simulink model "cog"  (R2025b)
settings: Solver=FixedStepAuto  StartTime=0.0  StopTime=10.0  FixedStep=0.01  RelTol=1e-3
libraries: matrix_library x3, SignalEditorBlockLib x1
settings Model: Creator=12482  LastModifiedBy=12482

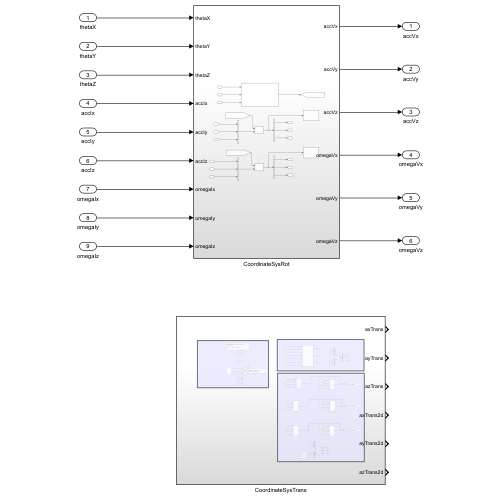
[thumbnail: Simulink's stored preview of the top-level diagram]
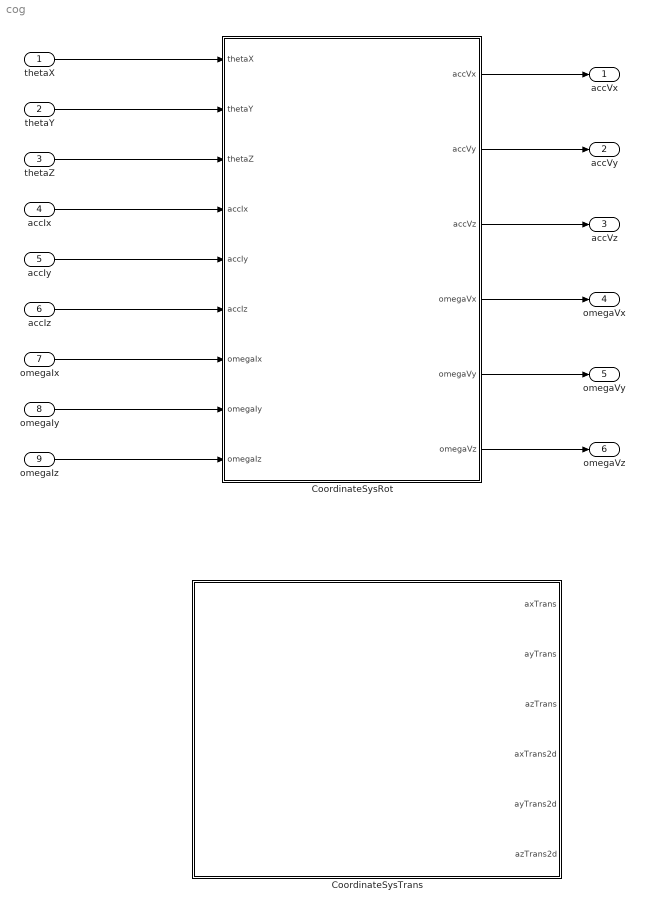
== system cog ==
  thetaX : Inport
  thetaY : Inport  Port=2
  thetaZ : Inport  Port=3
  accIx : Inport  Port=4
  accIy : Inport  Port=5
  accIz : Inport  Port=6
  omegaIx : Inport  Port=7
  omegaIy : Inport  Port=8
  omegaIz : Inport  Port=9
  CoordinateSysRot : Subsystem
  CoordinateSysTrans : Subsystem
  accVx : Outport
  accVy : Outport  Port=2
  accVz : Outport  Port=3
  omegaVx : Outport  Port=4
  omegaVy : Outport  Port=5
  omegaVz : Outport  Port=6
  wires:
  thetaX/1 -> CoordinateSysRot/1(thetaX)
  thetaY/1 -> CoordinateSysRot/2(thetaY)
  thetaZ/1 -> CoordinateSysRot/3(thetaZ)
  accIx/1 -> CoordinateSysRot/4(accIx)
  accIy/1 -> CoordinateSysRot/5(accIy)
  accIz/1 -> CoordinateSysRot/6(accIz)
  omegaIx/1 -> CoordinateSysRot/7(omegaIx)
  omegaIy/1 -> CoordinateSysRot/8(omegaIy)
  omegaIz/1 -> CoordinateSysRot/9(omegaIz)
  CoordinateSysRot/1(accVx) -> accVx/1
  CoordinateSysRot/2(accVy) -> accVy/1
  CoordinateSysRot/3(accVz) -> accVz/1
  CoordinateSysRot/4(omegaVx) -> omegaVx/1
  CoordinateSysRot/5(omegaVy) -> omegaVy/1
  CoordinateSysRot/6(omegaVz) -> omegaVz/1

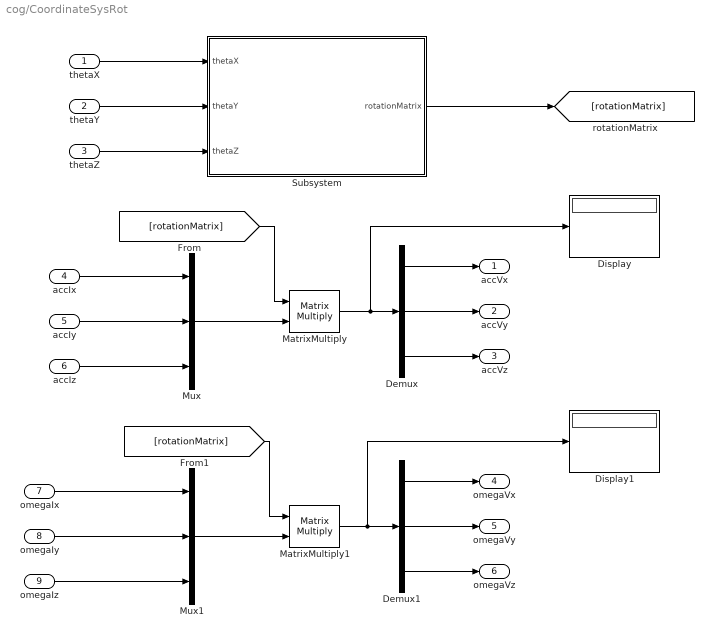
== system cog/CoordinateSysRot ==
  thetaX : Inport
  thetaY : Inport  Port=2
  thetaZ : Inport  Port=3
  accIx : Inport  Port=4
  accIy : Inport  Port=5
  accIz : Inport  Port=6
  omegaIx : Inport  Port=7
  omegaIy : Inport  Port=8
  omegaIz : Inport  Port=9
  Demux : Demux  Outputs=3
  Demux1 : Demux  Outputs=3
  Display : Display
  Display1 : Display
  MatrixMultiply : Product  Multiplication=Matrix(*)
  MatrixMultiply1 : Product  Multiplication=Matrix(*)
  Mux : Mux  Inputs=3
  Mux1 : Mux  Inputs=3
  Subsystem : Subsystem
  accVx : Outport
  accVy : Outport  Port=2
  accVz : Outport  Port=3
  omegaVx : Outport  Port=4
  omegaVy : Outport  Port=5
  omegaVz : Outport  Port=6
  wires:
  thetaX/1 -> Subsystem/1(thetaX)
  Demux1/3 -> omegaVz/1
  accIz/1 -> Mux/3
  Mux/1 -> MatrixMultiply/2
  thetaY/1 -> Subsystem/2(thetaY)
  MatrixMultiply/1 -> Display/1, Demux/1
  Subsystem/1(rotationMatrix) -> [rotationMatrix]
  thetaZ/1 -> Subsystem/3(thetaZ)
  Demux1/1 -> omegaVx/1
  accIx/1 -> Mux/1
  Demux1/2 -> omegaVy/1
  Demux/1 -> accVx/1
  accIy/1 -> Mux/2
  Demux/3 -> accVz/1
  Mux1/1 -> MatrixMultiply1/2
  [rotationMatrix] -> MatrixMultiply1/1
  omegaIx/1 -> Mux1/1
  omegaIy/1 -> Mux1/2
  MatrixMultiply1/1 -> Display1/1, Demux1/1
  [rotationMatrix] -> MatrixMultiply/1
  Demux/2 -> accVy/1
  omegaIz/1 -> Mux1/3

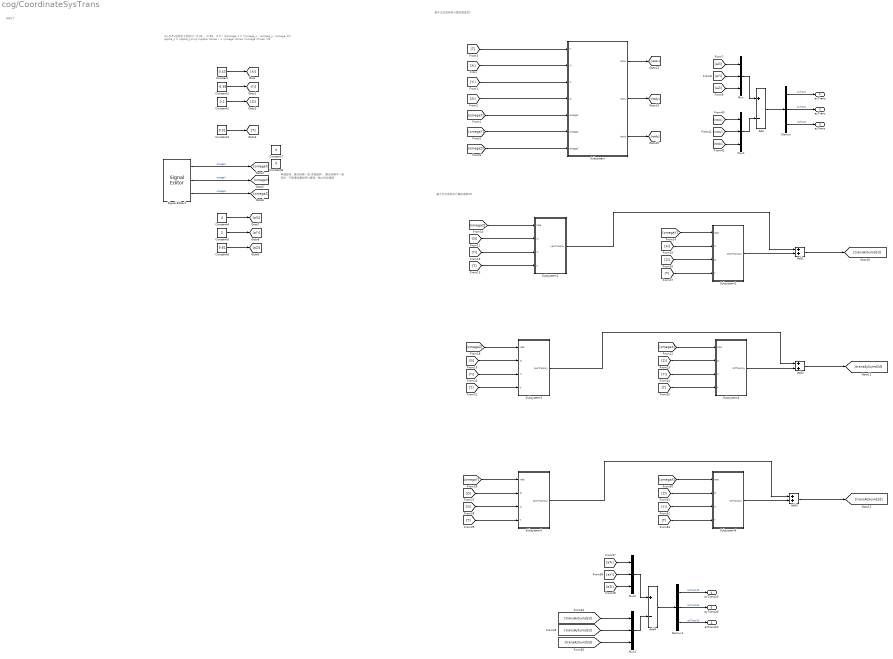
== system cog/CoordinateSysTrans ==
  note: 基于正交坐标系计算加速度2D
  note: 基于正交坐标系计算加速度3D
  note: INPUT
  note: 单轴旋转，算法结果一致
      | 多轴旋转， 算法结果不一致
      |
      | 结论：不能通过叠加来计算某一轴上的加速度
  note: imu在Rv坐标系下坐标为（0.43， -0.38， 0.2）
      | $\omega_c = (\omega_x, \omega_y, \omega_z)\\ \alpha_c = \alpha_{imu}-(\alpha \times r + \omega \times (\omega \times r))$
  Add : Sum  Inputs=+-
  Add1 : Sum
  Add2 : Sum
  Add3 : Sum
  Add4 : Sum  Inputs=+-
  Constant : Constant  Value=0.43
  Constant1 : Constant  Value=-0.38
  Constant2 : Constant  Value=0.2
  Constant3 : Constant  Value=0.01
  Constant4 : Constant  Value=4
  Constant5 : Constant  Value=2
  Constant6 : Constant  Value=9.81
  Constant7 : Constant  Value=0
  Constant8 : Constant  Value=0
  Demux : Demux  Outputs=3
  Demux1 : Demux  Outputs=3
  Mux{,1..3} (4 alike) : Mux  Inputs=3
  Signal Editor1 : SignalEditorBlockLib/Signal Editor  FileName=omega.mat  ActiveScenario=Scenario  ActiveSignal=omegaX  IsBus=off  OutputBusObjectStr=Bus: BusObject  SampleTime=0  ZeroCross=off  OutputAfterFinalValue=Setting to zero  Unit=inherit  PreserveSignalName=on  ApplySigPropsToAllScenarios=on  ApplySigPropsToAllSignals=on  SignalPropertySource=Dialog parameters
  Subsystem : Subsystem
  Subsystem1 : Subsystem
  Subsystem2 : Subsystem
  Subsystem3 : Subsystem
  Subsystem4 : Subsystem
  Subsystem5 : Subsystem
  Subsystem6 : Subsystem
  axTrans : Outport
  ayTrans : Outport  Port=2
  azTrans : Outport  Port=3
  axTrans2d : Outport  Port=4
  ayTrans2d : Outport  Port=5
  azTrans2d : Outport  Port=6
  wires:
  Constant4/1 -> [aXi]
  Constant5/1 -> [aYi]
  Constant6/1 -> [aZi]
  Constant/1 -> [Xi]
  Constant1/1 -> [Yi]
  Constant2/1 -> [Zi]
  Constant3/1 -> [T]
  [aXi] -> Mux/1
  [aYi] -> Mux/2
  [aZi] -> Mux/3
  Mux/1 -> Add/1
  Add/1 -> Demux/1
  Mux1/1 -> Add/2
  [omegaX] -> Subsystem/5(omegaX)
  [Zi] -> Subsystem/4(Zi)
  [omegaY] -> Subsystem/6(omegaY)
  [Yi] -> Subsystem/3(Yi)
  [omegaZ] -> Subsystem/7(omegaZ)
  [Xi] -> Subsystem/2(Xi)
  [T] -> Subsystem/1(T)
  Demux/2 -> ayTrans/1  "ayTrans"
  Demux/1 -> axTrans/1  "axTrans"
  Demux/3 -> azTrans/1  "azTrans"
  [Xi] -> Subsystem1/2(Xi)
  [Yi] -> Subsystem1/3(Yi)
  [omegaZ] -> Subsystem1/1(rate)
  [T] -> Subsystem1/4(T)
  [Xi] -> Subsystem2/2(Xi)
  [Zi] -> Subsystem2/3(Zi)
  [omegaY] -> Subsystem2/1(rate)
  [T] -> Subsystem2/4(T)
  [T] -> Subsystem3/4(T)
  [Xi] -> Subsystem3/2(Xi)
  [Yi] -> Subsystem3/3(Yi)
  [omegaZ] -> Subsystem3/1(rate)
  [T] -> Subsystem4/4(T)
  [Zi] -> Subsystem4/2(Zi)
  [Yi] -> Subsystem4/3(Yi)
  [omegaX] -> Subsystem4/1(rate)
  [T] -> Subsystem5/4(T)
  [omegaY] -> Subsystem5/1(rate)
  [Zi] -> Subsystem5/2(Zi)
  [Xi] -> Subsystem5/3(Xi)
  [T] -> Subsystem6/4(T)
  [Zi] -> Subsystem6/2(Zi)
  [Yi] -> Subsystem6/3(Yi)
  [omegaX] -> Subsystem6/1(rate)
  Subsystem1/1(yawTransAx) -> Add1/1
  Subsystem2/1(pitchTransAx) -> Add1/2
  Add1/1 -> [transAxSumd2d]
  Add2/1 -> [transAySumd2d]
  Add3/1 -> [transAzSumd2d]
  Subsystem6/1(rollTransAy) -> Add3/2
  Subsystem4/1(rollTransAy) -> Add2/2
  Subsystem3/1(yawTransAy) -> Add2/1
  Subsystem5/1(pitchTransAz) -> Add3/1
  Add4/1 -> Demux1/1
  Mux2/1 -> Add4/1
  [aXi] -> Mux2/1
  Mux3/1 -> Add4/2
  Demux1/3 -> azTrans2d/1  "azTrans2d"
  Demux1/1 -> axTrans2d/1  "axTrans2d"
  Demux1/2 -> ayTrans2d/1  "ayTrans2d"
  [aZi] -> Mux2/3
  [aYi] -> Mux2/2
  [transAzSumd2d] -> Mux3/3
  [transAySumd2d] -> Mux3/2
  [transAxSumd2d] -> Mux3/1
  Signal Editor1/1 -> [omegaX]  "omegaX"
  Signal Editor1/2 -> [omegaY]  "omegaY"
  Signal Editor1/3 -> [omegaZ]  "omegaZ"
  [rotAz] -> Mux1/3
  [rotAy] -> Mux1/2
  [rotAx] -> Mux1/1
  Subsystem/1(rotAx) -> [rotAx]
  Subsystem/2(rotAy) -> [rotAy]
  Subsystem/3(rotAz) -> [rotAz]

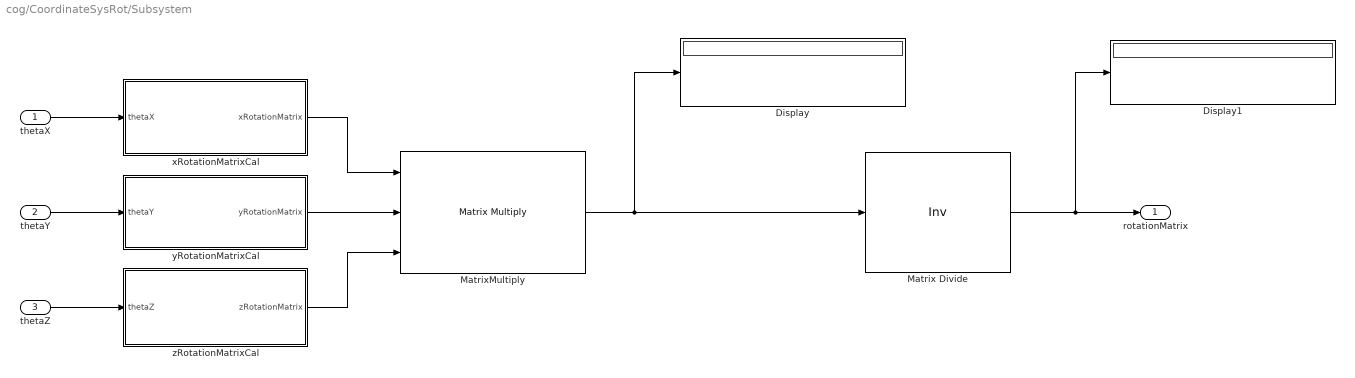
== system cog/CoordinateSysRot/Subsystem ==
  thetaX : Inport
  thetaY : Inport  Port=2
  thetaZ : Inport  Port=3
  Display : Display
  Display1 : Display
  Matrix Divide : Product  Inputs=/  Multiplication=Matrix(*)
  MatrixMultiply : Product  Inputs=3  Multiplication=Matrix(*)
  xRotationMatrixCal : MATLAB Function  TreatAsAtomicUnit=on
  yRotationMatrixCal : MATLAB Function  TreatAsAtomicUnit=on
  zRotationMatrixCal : MATLAB Function  TreatAsAtomicUnit=on
  rotationMatrix : Outport
  wires:
  zRotationMatrixCal/1(zRotationMatrix) -> MatrixMultiply/3
  thetaZ/1 -> zRotationMatrixCal/1(thetaZ)
  xRotationMatrixCal/1(xRotationMatrix) -> MatrixMultiply/1
  yRotationMatrixCal/1(yRotationMatrix) -> MatrixMultiply/2
  MatrixMultiply/1 -> Display/1, Matrix Divide/1
  thetaX/1 -> xRotationMatrixCal/1(thetaX)
  Matrix Divide/1 -> rotationMatrix/1, Display1/1
  thetaY/1 -> yRotationMatrixCal/1(thetaY)

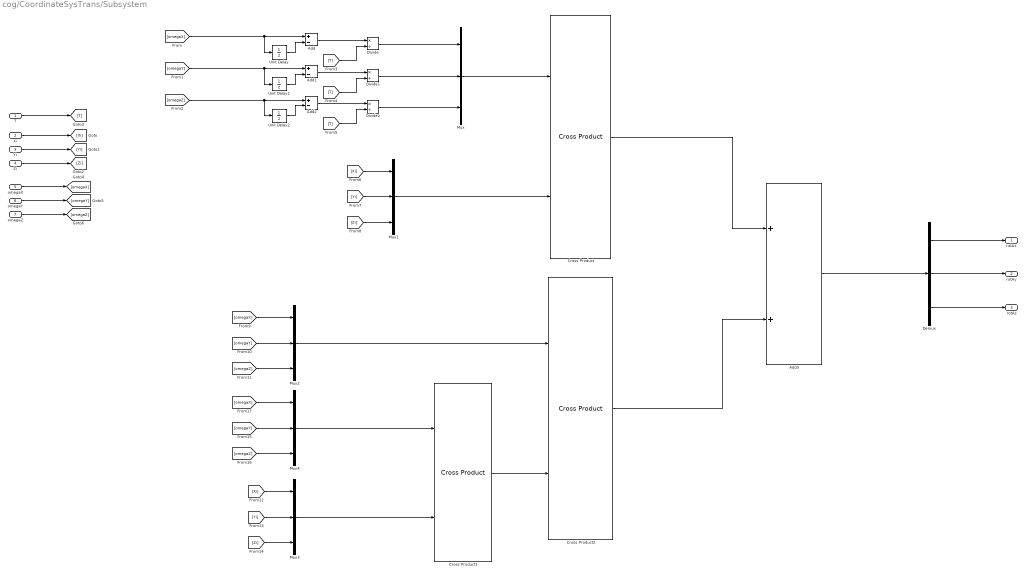
== system cog/CoordinateSysTrans/Subsystem ==
  T : Inport
  Xi : Inport  Port=2
  Yi : Inport  Port=3
  Zi : Inport  Port=4
  omegaX : Inport  Port=5
  omegaY : Inport  Port=6
  omegaZ : Inport  Port=7
  Add : Sum  Inputs=+-
  Add1 : Sum  Inputs=+-
  Add2 : Sum  Inputs=+-
  Add3 : Sum
  Cross Product : matrix_library/Cross Product
  Cross Product1 : matrix_library/Cross Product
  Cross Product2 : matrix_library/Cross Product
  Demux : Demux  Outputs=3
  Divide : Product  Inputs=*/
  Divide1 : Product  Inputs=*/
  Divide2 : Product  Inputs=*/
  Mux{,1..4} (5 alike) : Mux  Inputs=3
  Unit Delay : UnitDelay  SampleTime=-1  HasFrameUpgradeWarning=on
  Unit Delay1 : UnitDelay  SampleTime=-1  HasFrameUpgradeWarning=on
  Unit Delay2 : UnitDelay  SampleTime=-1  HasFrameUpgradeWarning=on
  rotAx : Outport
  rotAy : Outport  Port=2
  rotAz : Outport  Port=3
  wires:
  T/1 -> [T]
  Xi/1 -> [Xi]
  Yi/1 -> [Yi]
  Zi/1 -> [Zi]
  omegaX/1 -> [omegaX]
  omegaY/1 -> [omegaY]
  omegaZ/1 -> [omegaZ]
  [omegaX] -> Unit Delay/1, Add/1
  Unit Delay/1 -> Add/2
  Add/1 -> Divide/1
  [T] -> Divide/2
  [T] -> Divide1/2
  Add1/1 -> Divide1/1
  Unit Delay1/1 -> Add1/2
  [omegaY] -> Add1/1, Unit Delay1/1
  [omegaZ] -> Unit Delay2/1, Add2/1
  Unit Delay2/1 -> Add2/2
  Add2/1 -> Divide2/1
  [T] -> Divide2/2
  Divide/1 -> Mux/1
  Divide1/1 -> Mux/2
  Divide2/1 -> Mux/3
  Mux/1 -> Cross Product/1
  [Xi] -> Mux1/1
  [Yi] -> Mux1/2
  [Zi] -> Mux1/3
  Mux1/1 -> Cross Product/2
  Cross Product/1 -> Add3/1
  Add3/1 -> Demux/1
  Demux/3 -> rotAz/1
  Demux/2 -> rotAy/1
  Demux/1 -> rotAx/1
  [omegaY] -> Mux2/2
  [omegaX] -> Mux2/1
  [omegaZ] -> Mux2/3
  [Zi] -> Mux3/3
  [Yi] -> Mux3/2
  [Xi] -> Mux3/1
  [omegaZ] -> Mux4/3
  [omegaX] -> Mux4/1
  [omegaY] -> Mux4/2
  Mux4/1 -> Cross Product1/1
  Mux3/1 -> Cross Product1/2
  Mux2/1 -> Cross Product2/1
  Cross Product1/1 -> Cross Product2/2
  Cross Product2/1 -> Add3/2

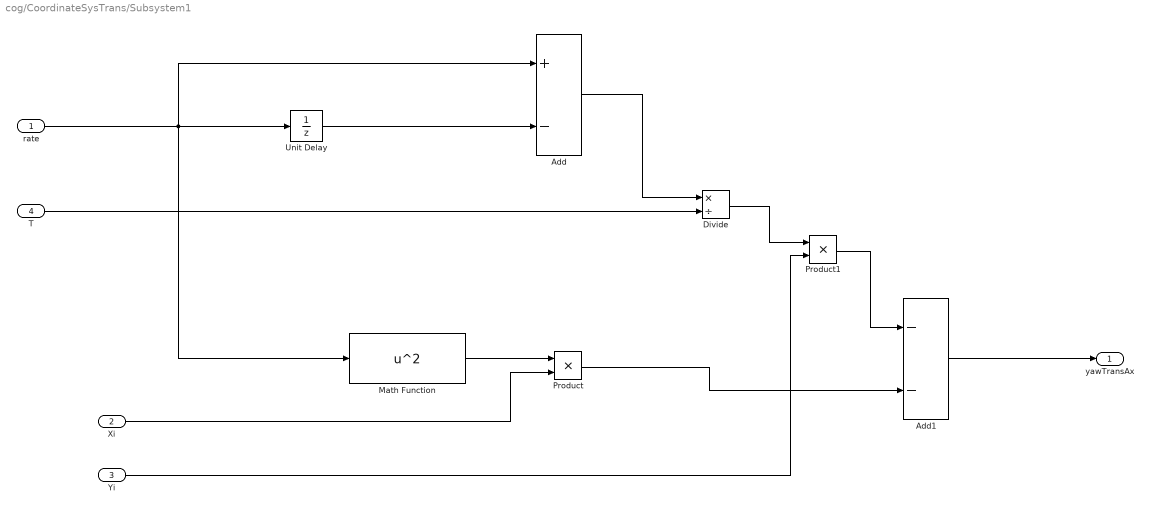
== system cog/CoordinateSysTrans/Subsystem1 ==
  rate : Inport
  Xi : Inport  Port=2
  Yi : Inport  Port=3
  T : Inport  Port=4
  Add : Sum  Inputs=+-
  Add1 : Sum  Inputs=--
  Divide : Product  Inputs=*/
  Math Function : Math  Operator=square
  Product : Product
  Product1 : Product
  Unit Delay : UnitDelay  SampleTime=-1  HasFrameUpgradeWarning=on
  yawTransAx : Outport
  wires:
  rate/1 -> Math Function/1, Add/1, Unit Delay/1
  Unit Delay/1 -> Add/2
  Add/1 -> Divide/1
  T/1 -> Divide/2
  Math Function/1 -> Product/1
  Divide/1 -> Product1/1
  Add1/1 -> yawTransAx/1
  Product/1 -> Add1/2
  Yi/1 -> Product1/2
  Product1/1 -> Add1/1
  Xi/1 -> Product/2

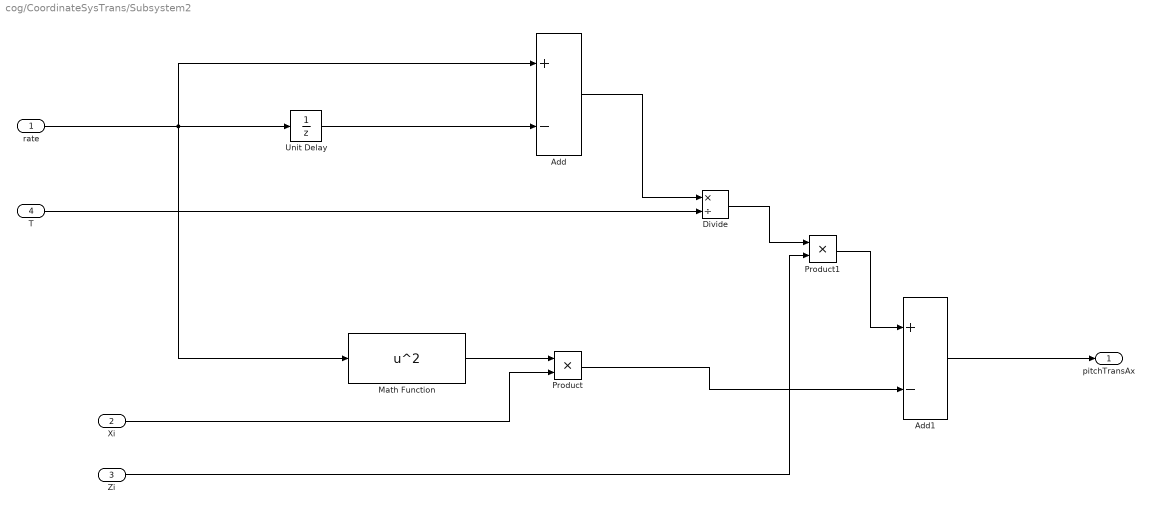
== system cog/CoordinateSysTrans/Subsystem2 ==
  rate : Inport
  Xi : Inport  Port=2
  Zi : Inport  Port=3
  T : Inport  Port=4
  Add : Sum  Inputs=+-
  Add1 : Sum  Inputs=+-
  Divide : Product  Inputs=*/
  Math Function : Math  Operator=square
  Product : Product
  Product1 : Product
  Unit Delay : UnitDelay  SampleTime=-1  HasFrameUpgradeWarning=on
  pitchTransAx : Outport
  wires:
  Xi/1 -> Product/2
  Product1/1 -> Add1/1
  Zi/1 -> Product1/2
  Product/1 -> Add1/2
  Add1/1 -> pitchTransAx/1
  Divide/1 -> Product1/1
  Math Function/1 -> Product/1
  T/1 -> Divide/2
  Add/1 -> Divide/1
  Unit Delay/1 -> Add/2
  rate/1 -> Unit Delay/1, Add/1, Math Function/1

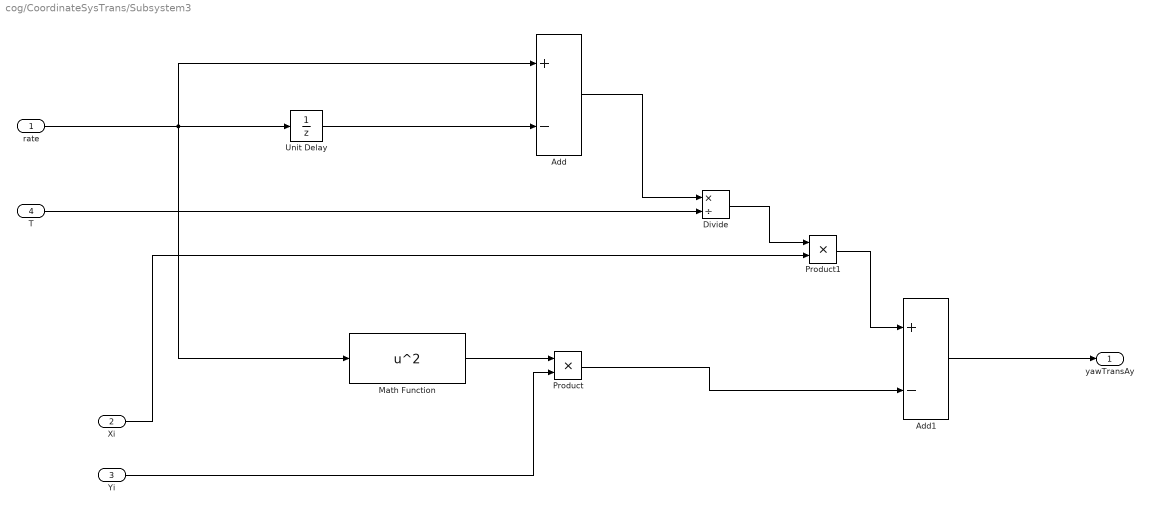
== system cog/CoordinateSysTrans/Subsystem3 ==
  rate : Inport
  Xi : Inport  Port=2
  Yi : Inport  Port=3
  T : Inport  Port=4
  Add : Sum  Inputs=+-
  Add1 : Sum  Inputs=+-
  Divide : Product  Inputs=*/
  Math Function : Math  Operator=square
  Product : Product
  Product1 : Product
  Unit Delay : UnitDelay  SampleTime=-1  HasFrameUpgradeWarning=on
  yawTransAy : Outport
  wires:
  Xi/1 -> Product1/2
  Product1/1 -> Add1/1
  Yi/1 -> Product/2
  Product/1 -> Add1/2
  Add1/1 -> yawTransAy/1
  Divide/1 -> Product1/1
  Math Function/1 -> Product/1
  T/1 -> Divide/2
  Add/1 -> Divide/1
  Unit Delay/1 -> Add/2
  rate/1 -> Unit Delay/1, Add/1, Math Function/1

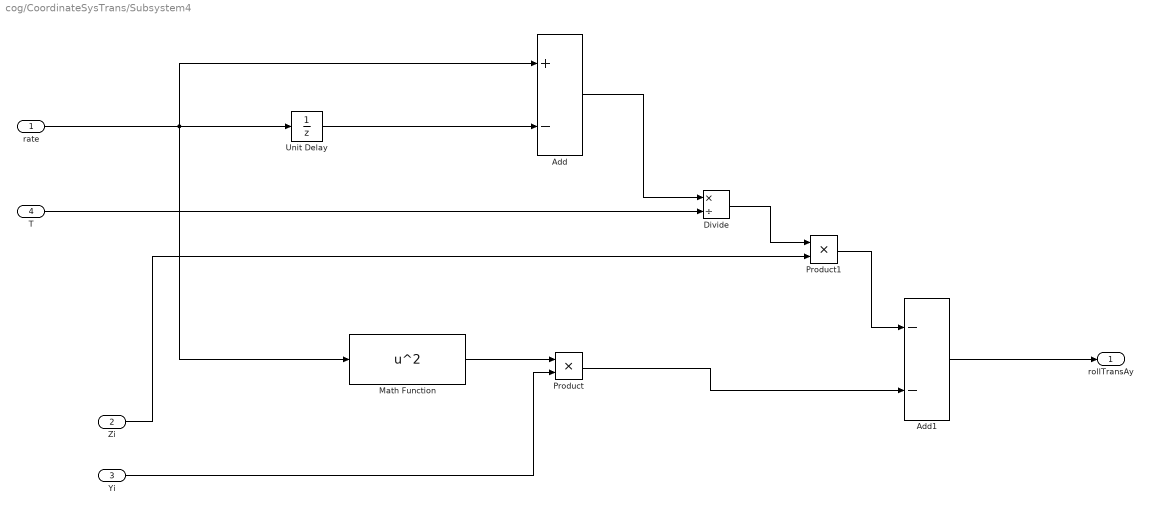
== system cog/CoordinateSysTrans/Subsystem4 ==
  rate : Inport
  Zi : Inport  Port=2
  Yi : Inport  Port=3
  T : Inport  Port=4
  Add : Sum  Inputs=+-
  Add1 : Sum  Inputs=--
  Divide : Product  Inputs=*/
  Math Function : Math  Operator=square
  Product : Product
  Product1 : Product
  Unit Delay : UnitDelay  SampleTime=-1  HasFrameUpgradeWarning=on
  rollTransAy : Outport
  wires:
  rate/1 -> Math Function/1, Add/1, Unit Delay/1
  Unit Delay/1 -> Add/2
  Add/1 -> Divide/1
  T/1 -> Divide/2
  Math Function/1 -> Product/1
  Divide/1 -> Product1/1
  Add1/1 -> rollTransAy/1
  Product/1 -> Add1/2
  Yi/1 -> Product/2
  Product1/1 -> Add1/1
  Zi/1 -> Product1/2

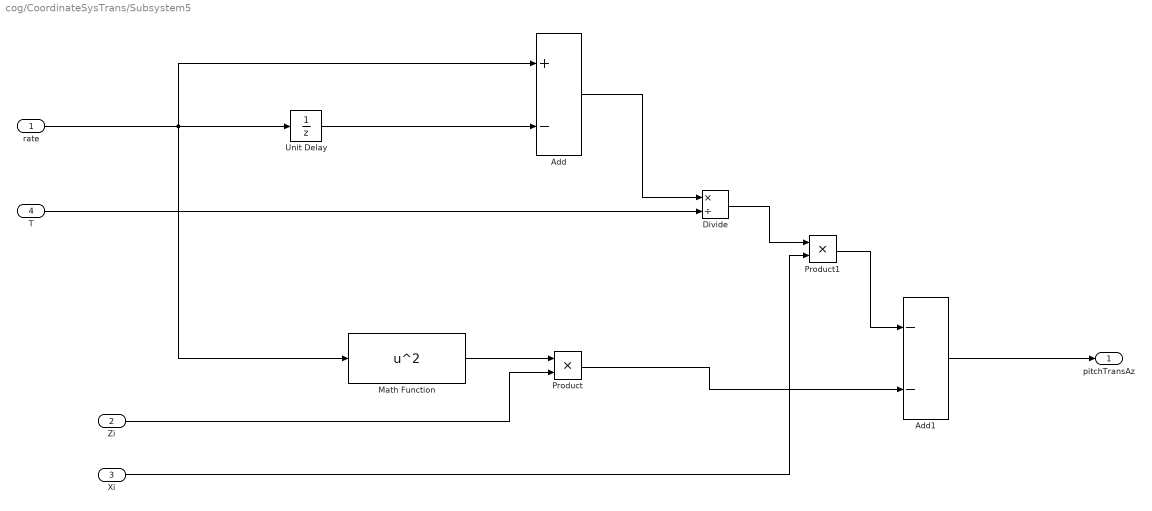
== system cog/CoordinateSysTrans/Subsystem5 ==
  rate : Inport
  Zi : Inport  Port=2
  Xi : Inport  Port=3
  T : Inport  Port=4
  Add : Sum  Inputs=+-
  Add1 : Sum  Inputs=--
  Divide : Product  Inputs=*/
  Math Function : Math  Operator=square
  Product : Product
  Product1 : Product
  Unit Delay : UnitDelay  SampleTime=-1  HasFrameUpgradeWarning=on
  pitchTransAz : Outport
  wires:
  rate/1 -> Math Function/1, Add/1, Unit Delay/1
  Unit Delay/1 -> Add/2
  Add/1 -> Divide/1
  T/1 -> Divide/2
  Math Function/1 -> Product/1
  Divide/1 -> Product1/1
  Add1/1 -> pitchTransAz/1
  Product/1 -> Add1/2
  Xi/1 -> Product1/2
  Product1/1 -> Add1/1
  Zi/1 -> Product/2

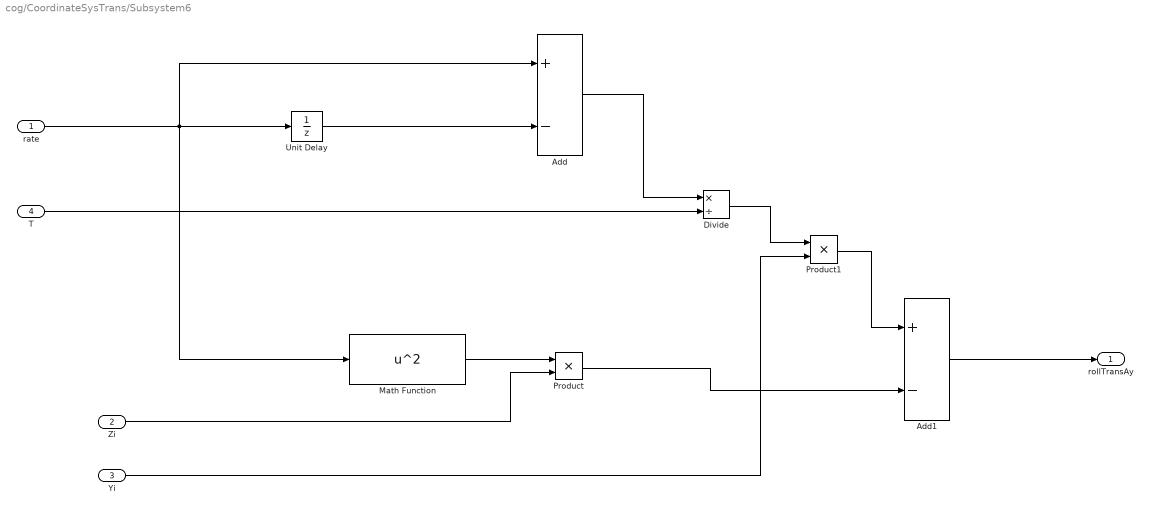
== system cog/CoordinateSysTrans/Subsystem6 ==
  rate : Inport
  Zi : Inport  Port=2
  Yi : Inport  Port=3
  T : Inport  Port=4
  Add : Sum  Inputs=+-
  Add1 : Sum  Inputs=+-
  Divide : Product  Inputs=*/
  Math Function : Math  Operator=square
  Product : Product
  Product1 : Product
  Unit Delay : UnitDelay  SampleTime=-1  HasFrameUpgradeWarning=on
  rollTransAy : Outport
  wires:
  Product1/1 -> Add1/1
  Product/1 -> Add1/2
  Add1/1 -> rollTransAy/1
  Divide/1 -> Product1/1
  Math Function/1 -> Product/1
  T/1 -> Divide/2
  Add/1 -> Divide/1
  Unit Delay/1 -> Add/2
  rate/1 -> Unit Delay/1, Add/1, Math Function/1
  Zi/1 -> Product/2
  Yi/1 -> Product1/2

== matlab function cog/CoordinateSysRot/Subsystem/xRotationMatrixCal ==
  data: thetaX input; xRotationMatrix output
function xRotationMatrix = xRotationMatrixCal(thetaX)
xMatrix = [1, 0, 0; 0, cos(thetaX), -sin(thetaX); 0, sin(thetaX), cos(thetaX)];
xRotationMatrix = xMatrix;

== matlab function cog/CoordinateSysRot/Subsystem/zRotationMatrixCal ==
  data: thetaZ input; zRotationMatrix output
function zRotationMatrix = zRotationMatrixCal(thetaZ)
zMatrix = [cos(thetaZ), -sin(thetaZ), 0; sin(thetaZ), cos(thetaZ), 0; 0, 0, 1];
zRotationMatrix = zMatrix;

== matlab function cog/CoordinateSysRot/Subsystem/yRotationMatrixCal ==
  data: thetaY input; yRotationMatrix output
function yRotationMatrix = yRotationMatrixCal(thetaY)
yMatrix = [cos(thetaY), 0, sin(thetaY); 0, 1, 0; -sin(thetaY), 0, cos(thetaY)];
yRotationMatrix = yMatrix;
